simulink model "Accel_model_test"  (R2016a)
settings: Solver=VariableStepAuto  StartTime=0.0  StopTime=5  RelTol=1e-3
values from neighbouring files (symbols this model uses):
  b = 0.5    [Initialisation_variables_workspace.m]    (also in TDNaccel.m = 0.0377358490566)
  C_mot = [0,45.126,51.01200000000001,52.974000000000004,51.01200000000001,48.069,49.050000000000004,51.01200000000001,56.898,58.86,58.86,57.879000000000005,56.898,54.936,51.993,48.069,44.145,40.221,36.297000000000004,32.373]    [Initialisation_variables_workspace.m]
  coeff_roul = 0.01    [Initialisation_variables_workspace.m]    (also in TDNaccel.m)
  Cx = 0.7    [Initialisation_variables_workspace.m]
  D_roue = 0.53    [Initialisation_variables_workspace.m]    (also in TDNaccel.m)
  e = 1.2    [Initialisation_variables_workspace.m]
  g = 9.81    [Initialisation_variables_workspace.m]    (also in TDNaccel.m)
  h = (mpilote*h_p + mveh*h_v)/m    (= 0.3)    [Initialisation_variables_workspace.m]
  J_eq = J_trans + 4*J_rot    (= 20.458125)    [Initialisation_variables_workspace.m]    (also in TDNaccel.m = 20.014125)
  m = mtot    (= 285)    [Initialisation_variables_workspace.m]    (also in TDNaccel.m)
  R = D_roue/2    (= 0.265)    [Initialisation_variables_workspace.m]    (also in TDNaccel.m = [R r])
  rap_couronne = 13/45    (= 0.288888888889)    [Initialisation_variables_workspace.m]
  rap_pri = 36/76    (= 0.473684210526)    [Initialisation_variables_workspace.m]
  regime = [0, 4500:500:13500]    [Initialisation_variables_workspace.m]
  rho = 1.2    [Initialisation_variables_workspace.m]
  S = 1    [Initialisation_variables_workspace.m]
  v = 1.2    [Initialisation_variables_workspace.m]    (also in TDNaccel.m = 0.133180615878)
  vitesse_initiale = 0    [Initialisation_variables_workspace.m]
undefined symbols (not defined in the file or in its folder): rap
settings Model: Creator=Aurélien  LastModifiedBy=Brice

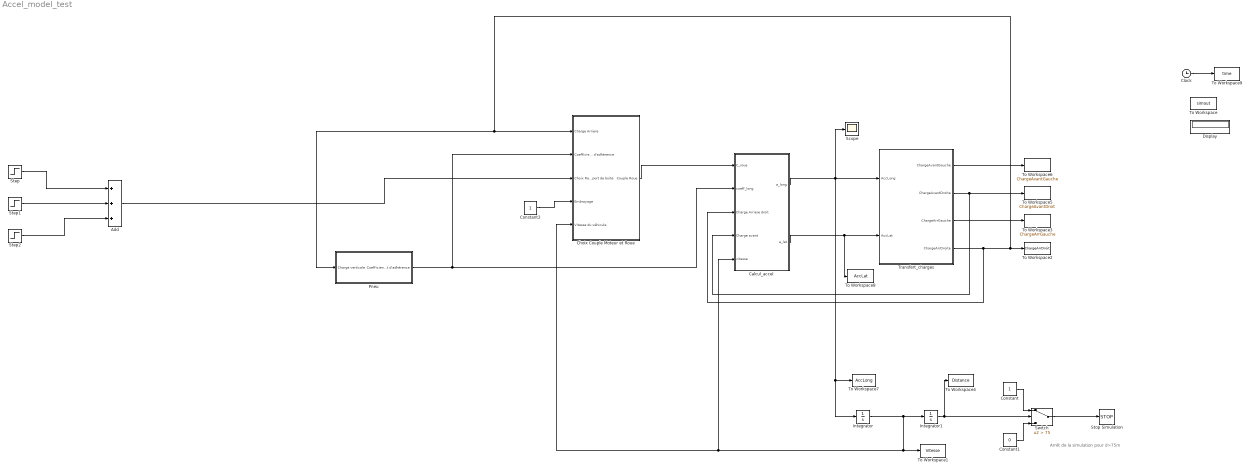
== system Accel_model_test ==
  note: Arrêt de la simulation pour d>75m
  Add : Sum  Inputs=+++
  Calcul_accel : Subsystem
  "Choix Couple Moteur et Roue " : Subsystem
  Clock : Clock
  Constant : Constant
  Constant1 : Constant  Value=0
  Constant2 : Constant
  Display : Display
  Integrator : Integrator
  Integrator1 : Integrator
  Pneu : Subsystem
  Scope : Scope
  Step : Step  Time=0  SampleTime=0
  Step1 : Step  Time=2  SampleTime=0
  Step2 : Step  Time=3  SampleTime=0
  Stop Simulation : Stop
  Switch : Switch  Criteria=u2 > Threshold  Threshold=75
  To Workspace : ToWorkspace  VariableName=simout  SaveFormat=Timeseries  SampleTime=-1
  To Workspace1 : ToWorkspace  VariableName=Vitesse  SaveFormat=Timeseries  SampleTime=-1
  To Workspace2 : ToWorkspace  VariableName=ChargeArrDroit  SaveFormat=Timeseries  SampleTime=-1
  To Workspace3 : ToWorkspace  VariableName=ChargeArrGauche  SaveFormat=Timeseries  SampleTime=-1
  To Workspace4 : ToWorkspace  VariableName=Distance  SaveFormat=Timeseries  SampleTime=-1
  To Workspace5 : ToWorkspace  VariableName=ChargeAvantDroit  SaveFormat=Timeseries  SampleTime=-1
  To Workspace6 : ToWorkspace  VariableName=ChargeAvantGauche  SaveFormat=Timeseries  SampleTime=-1
  To Workspace7 : ToWorkspace  VariableName=AccLong  SaveFormat=Timeseries  SampleTime=-1
  To Workspace8 : ToWorkspace  VariableName=AccLat  SaveFormat=Timeseries  SampleTime=-1
  To Workspace9 : ToWorkspace  VariableName=time  SampleTime=-1
  Transfert_charges : Subsystem
  wires:
  Integrator1/1 -> To Workspace4/1, Switch/2
  Switch/1 -> Stop Simulation/1
  Constant1/1 -> Switch/3
  Constant/1 -> Switch/1
  Integrator/1 -> Calcul_accel/5(vitesse), "Choix Couple Moteur et Roue "/5(Vitesse du véhicule), To Workspace1/1, Integrator1/1
  Transfert_charges/4(ChargeArrDroite) -> Calcul_accel/3("Charge Arriere droit "), Pneu/1(Charge verticale), "Choix Couple Moteur et Roue "/1(Charge Arriere), To Workspace2/1
  Transfert_charges/3(ChargeArrGauche) -> To Workspace3/1
  Transfert_charges/2(ChargeAvantDroite) -> Calcul_accel/4(Charge avant), To Workspace5/1
  Transfert_charges/1(ChargeAvantGauche) -> To Workspace6/1
  Calcul_accel/2(a_lat) -> To Workspace8/1, Transfert_charges/2(AccLat)
  Clock/1 -> To Workspace9/1
  "Choix Couple Moteur et Roue "/1(Couple Roue) -> Calcul_accel/1(C_roue)
  Pneu/1(Coefficient d'adhérence) -> Calcul_accel/2(coeff_long), "Choix Couple Moteur et Roue "/2("Coefficient d'adhérence ")
  Step/1 -> Add/1
  Calcul_accel/1(a_long) -> Integrator/1, To Workspace7/1, Scope/1, Transfert_charges/1(AccLong)
  Constant2/1 -> "Choix Couple Moteur et Roue "/4(Embrayage)
  Step1/1 -> Add/2
  Step2/1 -> Add/3
  Add/1 -> "Choix Couple Moteur et Roue "/3("Choix Rapport de boite ")

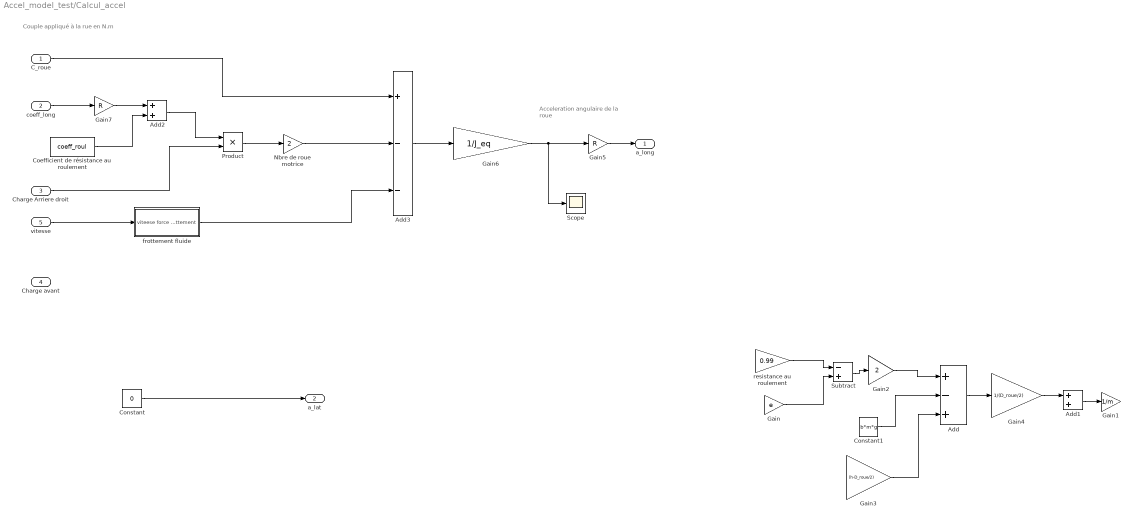
== system Accel_model_test/Calcul_accel ==
  note: Acceleration
      | angulaire
      | de la roue
  note: Couple appliqué à la rue en N.m
  C_roue : Inport
  coeff_long : Inport  Port=2
  "Charge Arriere droit " : Inport  Port=3
  Charge avant : Inport  Port=4
  vitesse : Inport  Port=5
  Add : Sum  Inputs=+-+
  Add1 : Sum
  Add2 : Sum
  Add3 : Sum  Inputs=+--
  Coefficient de résistance au roulement : Constant  Value=coeff_roul
  Constant : Constant  Value=0
  Constant1 : Constant  Value=b*m*g
  Gain : Gain  Gain=e
  Gain1 : Gain  Gain=1/m
  Gain2 : Gain  Gain=2
  Gain3 : Gain  Gain=(h-D_roue/2)
  Gain4 : Gain  Gain=1/(D_roue/2)
  Gain5 : Gain  Gain=R
  Gain6 : Gain  Gain=1/J_eq
  Gain7 : Gain  Gain=R
  Nbre de roue motrice : Gain  Gain=2
  Product : Product  Inputs=**
  Scope : Scope
  Subtract : Sum  Inputs=-+
  frottement fluide : Subsystem
  resistance au roulement : Gain  Gain=0.99
  a_long : Outport
  a_lat : Outport  Port=2
  wires:
  Constant/1 -> a_lat/1
  Gain/1 -> Subtract/2
  Subtract/1 -> Gain2/1
  resistance au roulement/1 -> Subtract/1
  Gain2/1 -> Add/1
  Constant1/1 -> Add/2
  Gain3/1 -> Add/3
  Add/1 -> Gain4/1
  Gain4/1 -> Add1/1
  Add1/1 -> Gain1/1
  Gain5/1 -> a_long/1
  Gain6/1 -> Scope/1, Gain5/1
  vitesse/1 -> frottement fluide/1(viteese)
  Gain7/1 -> Add2/1
  Coefficient de résistance au roulement/1 -> Add2/2
  Add2/1 -> Product/1
  coeff_long/1 -> Gain7/1
  "Charge Arriere droit "/1 -> Product/2
  Product/1 -> Nbre de roue motrice/1
  C_roue/1 -> Add3/1
  Nbre de roue motrice/1 -> Add3/2
  frottement fluide/1(force frottement) -> Add3/3
  Add3/1 -> Gain6/1

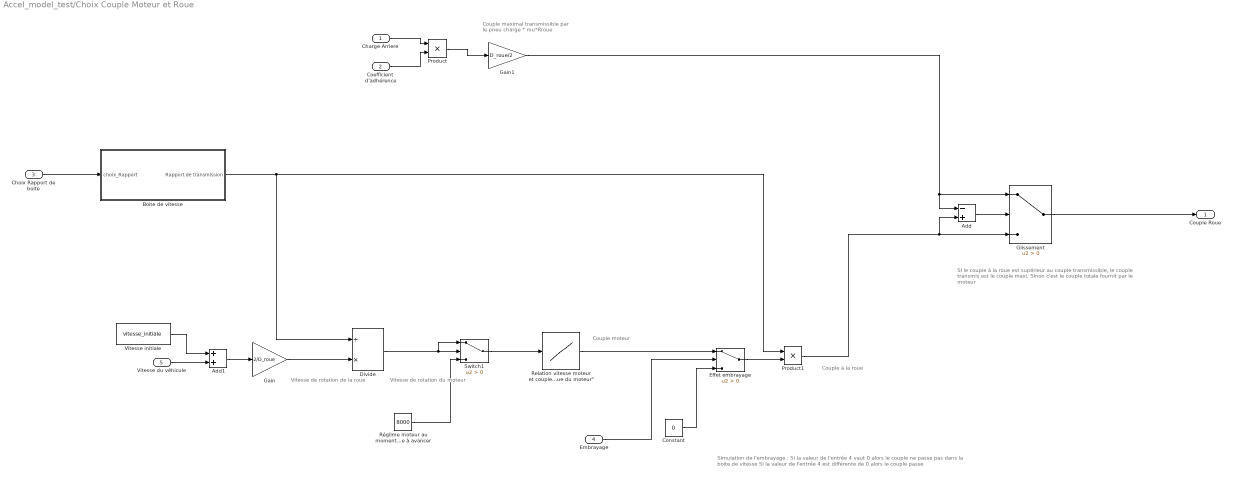
== system Accel_model_test/Choix Couple Moteur et Roue  ==
  note: Simulation de l'embrayage :
      | Si la valeur de l'entrée 4 vaut 0 alors le couple ne passe pas dans la boite de vitesse
      | Si la valeur de l'entrée 4 est différente de 0 alors le couple passe
  note: Vitesse de rotation
      | du moteur
  note: SI le couple à la roue est supérieur
      | au couple transmissible, le couple transmis est le couple maxi.
      | Sinon c'est le couple totale fournit par le moteur
  note: Couple à la roue
  note: Couple moteur
  note: Vitesse de rotation
      | de la roue
  note: Couple maximal transmissible
      | par le pneu charge * mu*Rroue
  Charge Arriere : Inport
  "Coefficient d'adhérence " : Inport  Port=2
  "Choix Rapport de boite " : Inport  Port=3
  Embrayage : Inport  Port=4
  Vitesse du véhicule : Inport  Port=5
  Add : Sum  Inputs=-+
  Add1 : Sum
  Boite de vitesse : Subsystem
  Constant : Constant  Value=0
  Divide : Product  Inputs=/*
  Effet embrayage : Switch  Criteria=u2 > Threshold
  Gain : Gain  Gain=2/D_roue
  Gain1 : Gain  Gain=D_roue/2
  Glissement : Switch  Criteria=u2 > Threshold
  Product : Product
  Product1 : Product
  "Relation vitesse moteur et couple moteur \"Caractéristique du moteur\"" : Lookup_n-D  NumberOfTableDimensions=1  BreakpointsForDimension1=regime  Table=C_mot  InternalRulePriority=Speed  RndMeth=Simplest  InputSameDT=on
  Régilme moteur au moment où le véhicule commence à avancer : Constant  Value=8000
  Switch1 : Switch  Criteria=u2 > Threshold
  Vitesse initiale : Constant  Value=vitesse_initiale
  Couple Roue : Outport
  wires:
  Vitesse du véhicule/1 -> Add1/2
  Vitesse initiale/1 -> Add1/1
  Add/1 -> Glissement/2
  "Choix Rapport de boite "/1 -> Boite de vitesse/1(choix_Rapport)
  Charge Arriere/1 -> Product/1
  "Coefficient d'adhérence "/1 -> Product/2
  Add1/1 -> Gain/1
  Product/1 -> Gain1/1
  Gain1/1 -> Add/1, Glissement/1
  Boite de vitesse/1(Rapport de transmission) -> Divide/1, Product1/1
  Product1/1 -> Add/2, Glissement/3
  Glissement/1 -> Couple Roue/1
  Gain/1 -> Divide/2
  Divide/1 -> Switch1/1, Switch1/2
  Régilme moteur au moment où le véhicule commence à avancer/1 -> Switch1/3
  Switch1/1 -> "Relation vitesse moteur et couple moteur \"Caractéristique du moteur\""/1
  "Relation vitesse moteur et couple moteur \"Caractéristique du moteur\""/1 -> Effet embrayage/1
  Effet embrayage/1 -> Product1/2
  Constant/1 -> Effet embrayage/3
  Embrayage/1 -> Effet embrayage/2

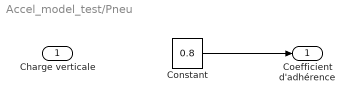
== system Accel_model_test/Pneu ==
  Charge verticale : Inport
  Constant : Constant  Value=0.8
  Coefficient d'adhérence : Outport
  wires:
  Constant/1 -> Coefficient d'adhérence/1

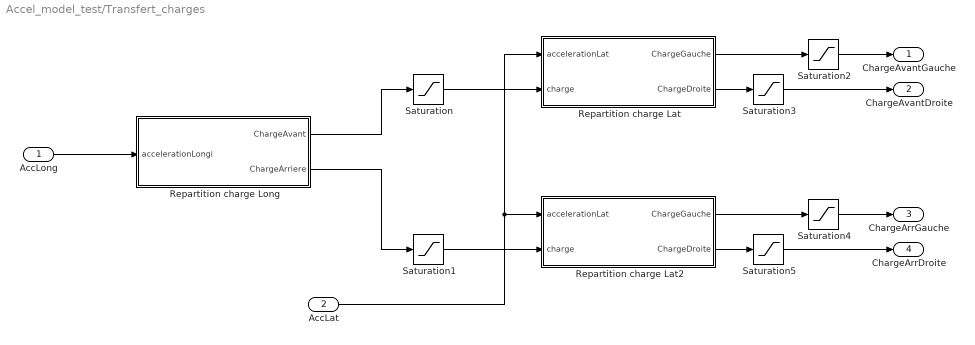
== system Accel_model_test/Transfert_charges ==
  AccLong : Inport
  AccLat : Inport  Port=2
  Repartition charge Lat : Subsystem
  Repartition charge Lat2 : Subsystem
  Repartition charge Long : Subsystem
  Saturation : Saturate  UpperLimit=inf  LowerLimit=0
  Saturation{1..5} (5 alike) : Saturate  UpperLimit=m*g  LowerLimit=0
  ChargeAvantGauche : Outport
  ChargeAvantDroite : Outport  Port=2
  ChargeArrGauche : Outport  Port=3
  ChargeArrDroite : Outport  Port=4
  wires:
  Repartition charge Long/1(ChargeAvant) -> Saturation/1
  Repartition charge Long/2(ChargeArriere) -> Saturation1/1
  AccLong/1 -> Repartition charge Long/1(accelerationLongi)
  AccLat/1 -> Repartition charge Lat/1(accelerationLat), Repartition charge Lat2/1(accelerationLat)
  Repartition charge Lat/2(ChargeDroite) -> Saturation3/1
  Repartition charge Lat/1(ChargeGauche) -> Saturation2/1
  Repartition charge Lat2/1(ChargeGauche) -> Saturation4/1
  Repartition charge Lat2/2(ChargeDroite) -> Saturation5/1
  Saturation/1 -> Repartition charge Lat/2("charge ")
  Saturation1/1 -> Repartition charge Lat2/2("charge ")
  Saturation2/1 -> ChargeAvantGauche/1
  Saturation3/1 -> ChargeAvantDroite/1
  Saturation4/1 -> ChargeArrGauche/1
  Saturation5/1 -> ChargeArrDroite/1

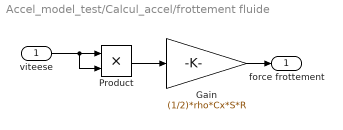
== system Accel_model_test/Calcul_accel/frottement fluide ==
  viteese : Inport
  Gain : Gain  Gain=(1/2)*rho*Cx*S*R
  Product : Product
  force frottement : Outport
  wires:
  viteese/1 -> Product/2, Product/1
  Gain/1 -> force frottement/1
  Product/1 -> Gain/1

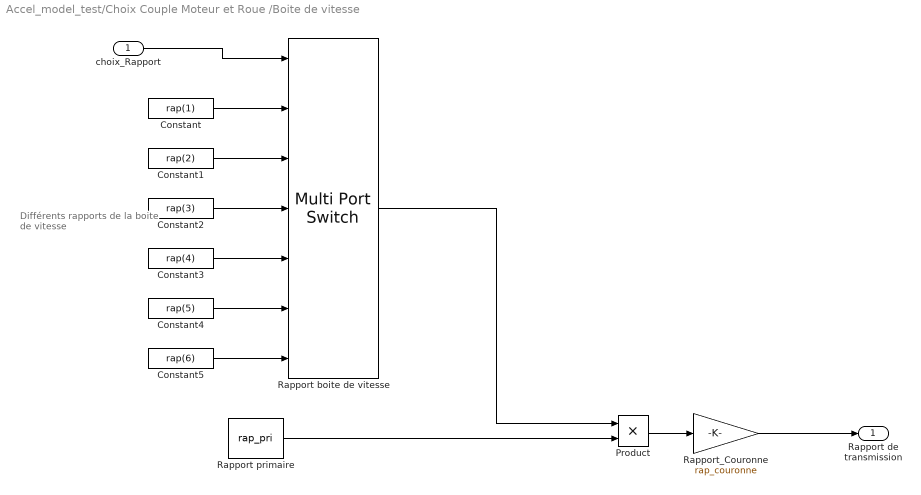
== system Accel_model_test/Choix Couple Moteur et Roue /Boite de vitesse ==
  note: Différents rapports
      | de la boite de vitesse
  choix_Rapport : Inport
  Constant : Constant  Value=rap(1)
  Constant1 : Constant  Value=rap(2)
  Constant2 : Constant  Value=rap(3)
  Constant3 : Constant  Value=rap(4)
  Constant4 : Constant  Value=rap(5)
  Constant5 : Constant  Value=rap(6)
  Product : Product
  Rapport primaire : Constant  Value=rap_pri
  Rapport boite de vitesse : MultiPortSwitch  Inputs=6
  Rapport_Couronne : Gain  Gain=rap_couronne
  Rapport de transmission : Outport
  wires:
  Constant/1 -> Rapport boite de vitesse/2
  Constant1/1 -> Rapport boite de vitesse/3
  Constant2/1 -> Rapport boite de vitesse/4
  Constant3/1 -> Rapport boite de vitesse/5
  Constant4/1 -> Rapport boite de vitesse/6
  choix_Rapport/1 -> Rapport boite de vitesse/1
  Rapport boite de vitesse/1 -> Product/1
  Rapport_Couronne/1 -> Rapport de transmission/1
  Product/1 -> Rapport_Couronne/1
  Rapport primaire/1 -> Product/2
  Constant5/1 -> Rapport boite de vitesse/7

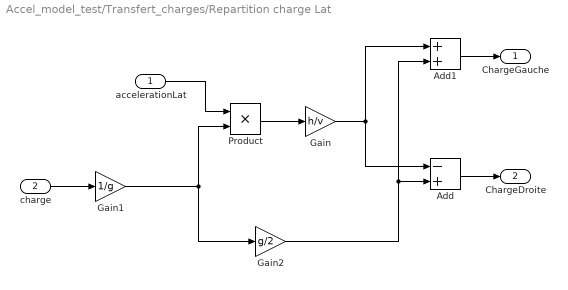
== system Accel_model_test/Transfert_charges/Repartition charge Lat ==
  accelerationLat : Inport
  "charge " : Inport  Port=2
  Add : Sum  Inputs=-+
  Add1 : Sum
  Gain : Gain  Gain=h/v
  Gain1 : Gain  Gain=1/g
  Gain2 : Gain  Gain=g/2
  Product : Product
  ChargeGauche : Outport
  ChargeDroite : Outport  Port=2
  wires:
  Gain/1 -> Add1/1, Add/1
  Add1/1 -> ChargeGauche/1
  Add/1 -> ChargeDroite/1
  accelerationLat/1 -> Product/1
  "charge "/1 -> Gain1/1
  Product/1 -> Gain/1
  Gain2/1 -> Add1/2, Add/2
  Gain1/1 -> Gain2/1, Product/2

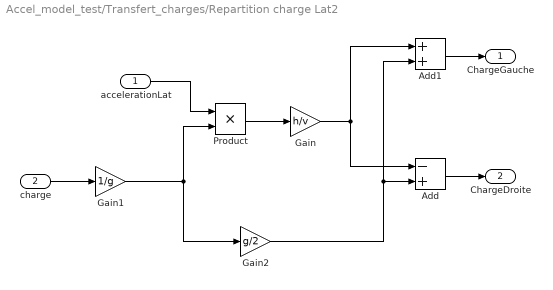
== system Accel_model_test/Transfert_charges/Repartition charge Lat2 ==
  accelerationLat : Inport
  "charge " : Inport  Port=2
  Add : Sum  Inputs=-+
  Add1 : Sum
  Gain : Gain  Gain=h/v
  Gain1 : Gain  Gain=1/g
  Gain2 : Gain  Gain=g/2
  Product : Product
  ChargeGauche : Outport
  ChargeDroite : Outport  Port=2
  wires:
  Gain/1 -> Add1/1, Add/1
  Add1/1 -> ChargeGauche/1
  Add/1 -> ChargeDroite/1
  accelerationLat/1 -> Product/1
  "charge "/1 -> Gain1/1
  Product/1 -> Gain/1
  Gain2/1 -> Add1/2, Add/2
  Gain1/1 -> Product/2, Gain2/1

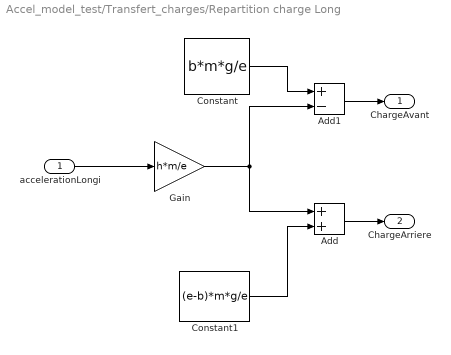
== system Accel_model_test/Transfert_charges/Repartition charge Long ==
  accelerationLongi : Inport
  Add : Sum
  Add1 : Sum  Inputs=+-
  Constant : Constant  Value=b*m*g/e
  Constant1 : Constant  Value=(e-b)*m*g/e
  Gain : Gain  Gain=h*m/e
  ChargeAvant : Outport
  ChargeArriere : Outport  Port=2
  wires:
  accelerationLongi/1 -> Gain/1
  Gain/1 -> Add/1, Add1/2
  Constant/1 -> Add1/1
  Constant1/1 -> Add/2
  Add1/1 -> ChargeAvant/1
  Add/1 -> ChargeArriere/1
